simulink model "Control"  (R2025b)
settings: Solver=ode4  StartTime=0.0  StopTime=10.0  FixedStep=0.01  RelTol=1e-3
undefined symbols (not defined in the file): Control_Force_Limit, Control_phasing_power_threshold, Control_saturation_power_threshold, Control_switch, d_pulse_frequency, Dynamic_Nav_Gain, Dynamic_Navigation_constant, m_mass, Nav_constant, Phasing_switch, Pure_Pursuit_Centered_angle_Z, Pure_Pursuit_Y_Gain, Pure_Pursuit_Z_Gain, Ref_speed, s_energy_threshold
libraries: simulink x3
settings Model: DataDictionary=Control_data.sldd  Creator=mauro  LastModifiedBy=mauro

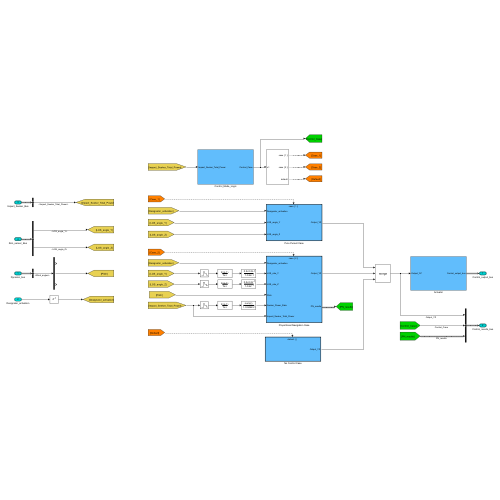
[thumbnail: Simulink's stored preview of the top-level diagram]
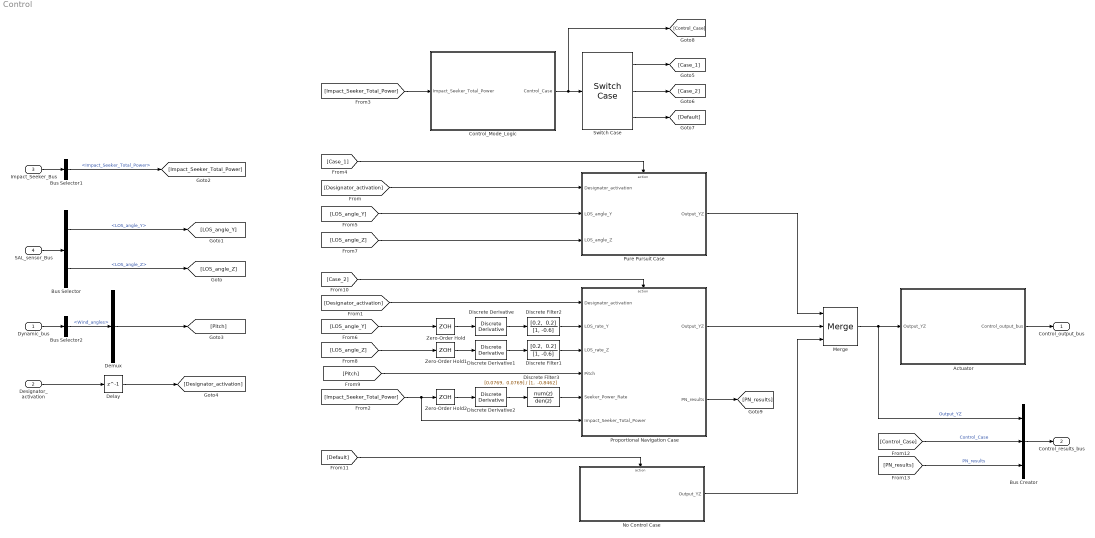
== system Control ==
  Dynamic_bus : Inport  OutDataTypeStr=Bus: Dynamic_bus
  Designator_activation : Inport  Port=2  OutDataTypeStr=double  SampleTime=0.01
  Impact_Seeker_Bus : Inport  Port=3  OutDataTypeStr=Bus: Impact_Seeker_Bus  BusOutputAsStruct=on
  SAL_sensor_Bus : Inport  Port=4  OutDataTypeStr=Bus: SAL_sensor_Bus  SampleTime=0.01  BusOutputAsStruct=on
  Actuator : Subsystem
  Bus Creator : BusCreator  Inputs=3  OutDataTypeStr=Bus: Control_results_bus  NonVirtualBus=on
  Bus Selector : BusSelector  OutputSignals=LOS_angle_Y,LOS_angle_Z
  Bus Selector1 : BusSelector  OutputSignals=Impact_Seeker_Total_Power
  Bus Selector2 : BusSelector  OutputSignals=Wind_angles
  Control_Mode_Logic : Subsystem
  Delay : Delay  DelayLength=1  InitialCondition=0
  Demux : Demux  Outputs=3
  Discrete Derivative : simulink/Discrete/Discrete Derivative  gainval=1.0  ICPrevScaledInput=0.0  OutMin=[]  OutMax=[]  OutDataType=fixdt(1, 16)  OutScaling=2^-10  DoSatur=off
  Discrete Derivative1 : simulink/Discrete/Discrete Derivative  gainval=1.0  ICPrevScaledInput=0  OutMin=[]  OutMax=[]  OutDataType=fixdt(1, 16)  OutScaling=2^-10  DoSatur=off
  Discrete Derivative2 : simulink/Discrete/Discrete Derivative  gainval=1.0  ICPrevScaledInput=0  OutMin=[]  OutMax=[]  OutDataType=fixdt(1, 16)  OutScaling=2^-10  DoSatur=off
  Discrete Filter1 : DiscreteFilter  Numerator="[0.2,  0.2]"  Denominator=[1, -0.6]
  Discrete Filter2 : DiscreteFilter  Numerator="[0.2,  0.2]"  Denominator=[1, -0.6]
  Discrete Filter3 : DiscreteFilter  Numerator="[0.0769,  0.0769]"  Denominator="[1,  -0.8462]"
  Merge : Merge  Inputs=3  InitialOutput=[0 0]
  No Control Case : Subsystem  TreatAsAtomicUnit=on
  Proportional Navigation Case : Subsystem  TreatAsAtomicUnit=on
  Pure Pursuit Case : Subsystem  TreatAsAtomicUnit=on
  Switch Case : SwitchCase  CaseConditions={1,2}
  Zero-Order Hold : ZeroOrderHold  SampleTime=1/d_pulse_frequency
  Zero-Order Hold1 : ZeroOrderHold  SampleTime=1/d_pulse_frequency
  Zero-Order Hold2 : ZeroOrderHold  SampleTime=1/d_pulse_frequency
  Control_output_bus : Outport  OutDataTypeStr=Bus: Control_output_bus  BusOutputAsStruct=on
  Control_results_bus : Outport  Port=2  OutDataTypeStr=Bus: Control_results_bus  BusOutputAsStruct=on
  wires:
  SAL_sensor_Bus/1 -> Bus Selector/1
  Bus Selector/2 -> [LOS_angle_Z]  "<LOS_angle_Z>"
  Bus Selector/1 -> [LOS_angle_Y]  "<LOS_angle_Y>"
  Dynamic_bus/1 -> Bus Selector2/1
  Bus Selector2/1 -> Demux/1  "<Wind_angles>"
  Actuator/1(Control_output_bus) -> Control_output_bus/1
  [Designator_activation] -> Pure Pursuit Case/1(Designator_activation)
  [Designator_activation] -> Proportional Navigation Case/1(Designator_activation)
  [LOS_angle_Y] -> Pure Pursuit Case/2(LOS_angle_Y)
  [LOS_angle_Z] -> Pure Pursuit Case/3(LOS_angle_Z)
  [Pitch] -> Proportional Navigation Case/4(Pitch)
  Proportional Navigation Case/1(Output_YZ) -> Merge/2
  Pure Pursuit Case/1(Output_YZ) -> Merge/1
  No Control Case/1(Output_YZ) -> Merge/3
  Merge/1 -> Bus Creator/1, Actuator/1(Output_YZ)  "Output_YZ"
  Control_Mode_Logic/1(Control_Case) -> [Control_Case], Switch Case/1
  Demux/2 -> [Pitch]
  Delay/1 -> [Designator_activation]
  Designator_activation/1 -> Delay/1
  [LOS_angle_Z] -> Zero-Order Hold1/1
  Discrete Derivative/1 -> Discrete Filter2/1
  Zero-Order Hold/1 -> Discrete Derivative/1
  [LOS_angle_Y] -> Zero-Order Hold/1
  Zero-Order Hold1/1 -> Discrete Derivative1/1
  Discrete Derivative1/1 -> Discrete Filter1/1
  Discrete Filter1/1 -> Proportional Navigation Case/3(LOS_rate_Z)
  Discrete Filter2/1 -> Proportional Navigation Case/2(LOS_rate_Y)
  Impact_Seeker_Bus/1 -> Bus Selector1/1
  Bus Selector1/1 -> [Impact_Seeker_Total_Power]  "<Impact_Seeker_Total_Power>"
  [Impact_Seeker_Total_Power] -> Control_Mode_Logic/1(Impact_Seeker_Total_Power)
  Zero-Order Hold2/1 -> Discrete Derivative2/1
  [Impact_Seeker_Total_Power] -> Zero-Order Hold2/1, Proportional Navigation Case/6(Impact_Seeker_Total_Power)
  Bus Creator/1 -> Control_results_bus/1
  Switch Case/1 -> [Case_1]
  Switch Case/2 -> [Case_2]
  Switch Case/3 -> [Default]
  [Case_1] -> Pure Pursuit Case/Action
  [Case_2] -> Proportional Navigation Case/Action
  [Default] -> No Control Case/Action
  Proportional Navigation Case/2(PN_results) -> [PN_results]
  [PN_results] -> Bus Creator/3  "PN_results"
  [Control_Case] -> Bus Creator/2  "Control_Case"
  Discrete Derivative2/1 -> Discrete Filter3/1
  Discrete Filter3/1 -> Proportional Navigation Case/5(Seeker_Power_Rate)

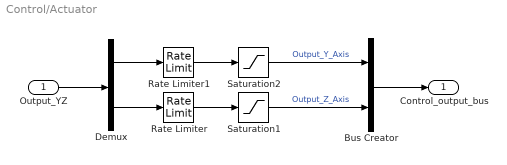
== system Control/Actuator ==
  Output_YZ : Inport
  Bus Creator : BusCreator  Inputs=2
  Demux : Demux  Outputs=2
  Rate Limiter : RateLimiter  RisingSlewLimit=1000  FallingSlewLimit=-1000  SampleTimeMode=inherited
  Rate Limiter1 : RateLimiter  RisingSlewLimit=2000  FallingSlewLimit=-2000  SampleTimeMode=inherited
  Saturation1 : Saturate  UpperLimit=Control_Force_Limit  LowerLimit=-Control_Force_Limit
  Saturation2 : Saturate  UpperLimit=Control_Force_Limit  LowerLimit=-Control_Force_Limit
  Control_output_bus : Outport  OutDataTypeStr=Bus: Control_output_bus
  wires:
  Saturation2/1 -> Bus Creator/1  "Output_Y_Axis"
  Rate Limiter1/1 -> Saturation2/1
  Output_YZ/1 -> Demux/1
  Saturation1/1 -> Bus Creator/2  "Output_Z_Axis"
  Bus Creator/1 -> Control_output_bus/1
  Rate Limiter/1 -> Saturation1/1
  Demux/1 -> Rate Limiter1/1
  Demux/2 -> Rate Limiter/1

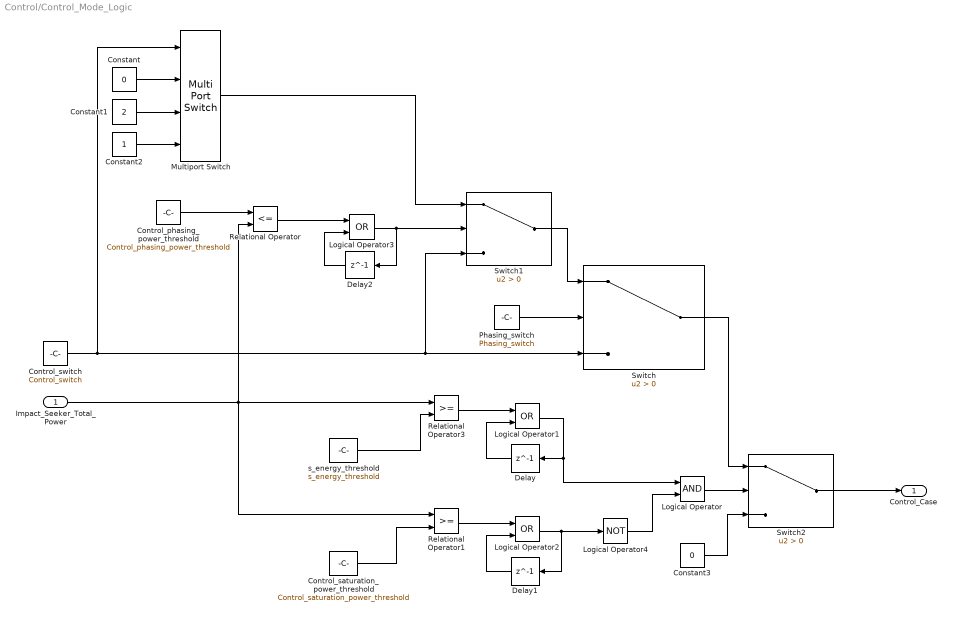
== system Control/Control_Mode_Logic ==
  Impact_Seeker_Total_Power : Inport
  Constant : Constant  Value=0
  Constant1 : Constant  Value=2
  Constant2 : Constant
  Constant3 : Constant  Value=0
  Control_phasing_power_threshold : Constant  Value=Control_phasing_power_threshold
  Control_saturation_power_threshold : Constant  Value=Control_saturation_power_threshold
  Control_switch : Constant  Value=Control_switch
  Delay : Delay  DelayLength=1  InitialCondition=0
  Delay1 : Delay  DelayLength=1  InitialCondition=0
  Delay2 : Delay  DelayLength=1  InitialCondition=0
  Logical Operator : Logic  AllPortsSameDT=off  OutDataTypeStr=boolean
  Logical Operator1 : Logic  Operator=OR  AllPortsSameDT=off  OutDataTypeStr=boolean
  Logical Operator2 : Logic  Operator=OR  AllPortsSameDT=off  OutDataTypeStr=boolean
  Logical Operator3 : Logic  Operator=OR  AllPortsSameDT=off  OutDataTypeStr=boolean
  Logical Operator4 : Logic  Operator=NOT  AllPortsSameDT=off  OutDataTypeStr=boolean
  Multiport Switch : MultiPortSwitch  DataPortOrder=Zero-based contiguous  zeroidx=on  SaturateOnIntegerOverflow=off  InputSameDT=off
  Phasing_switch : Constant  Value=Phasing_switch
  Relational Operator : RelationalOperator  Operator=<=  OutDataTypeStr=boolean  RndMeth=Simplest  InputSameDT=off
  Relational Operator1 : RelationalOperator  OutDataTypeStr=boolean  RndMeth=Simplest  InputSameDT=off
  Relational Operator3 : RelationalOperator  OutDataTypeStr=boolean  RndMeth=Simplest  InputSameDT=off
  Switch : Switch  Criteria=u2 > Threshold  SaturateOnIntegerOverflow=off  InputSameDT=off
  Switch1 : Switch  Criteria=u2 > Threshold  SaturateOnIntegerOverflow=off  InputSameDT=off
  Switch2 : Switch  Criteria=u2 > Threshold  SaturateOnIntegerOverflow=off  InputSameDT=off
  s_energy_threshold : Constant  Value=s_energy_threshold
  Control_Case : Outport
  wires:
  Control_switch/1 -> Switch/3, Switch1/3, Multiport Switch/1
  Switch1/1 -> Switch/1
  s_energy_threshold/1 -> Relational Operator3/2
  Phasing_switch/1 -> Switch/2
  Control_phasing_power_threshold/1 -> Relational Operator/1
  Switch/1 -> Switch2/1
  Constant3/1 -> Switch2/3
  Constant/1 -> Multiport Switch/2
  Constant2/1 -> Multiport Switch/4
  Multiport Switch/1 -> Switch1/1
  Constant1/1 -> Multiport Switch/3
  Switch2/1 -> Control_Case/1
  Logical Operator1/1 -> Logical Operator/1, Delay/1
  Relational Operator3/1 -> Logical Operator1/1
  Delay/1 -> Logical Operator1/2
  Logical Operator2/1 -> Delay1/1, Logical Operator4/1
  Delay1/1 -> Logical Operator2/2
  Relational Operator1/1 -> Logical Operator2/1
  Logical Operator3/1 -> Delay2/1, Switch1/2
  Delay2/1 -> Logical Operator3/2
  Relational Operator/1 -> Logical Operator3/1
  Control_saturation_power_threshold/1 -> Relational Operator1/2
  Logical Operator/1 -> Switch2/2
  Logical Operator4/1 -> Logical Operator/2
  Impact_Seeker_Total_Power/1 -> Relational Operator3/1, Relational Operator1/1, Relational Operator/2

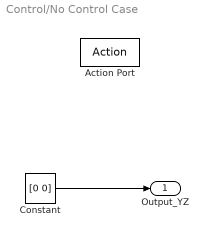
== system Control/No Control Case ==
  Action Port : ActionPort  ActionPortLabel=default:
  Constant : Constant  Value=[0 0]
  Output_YZ : Outport
  wires:
  Constant/1 -> Output_YZ/1

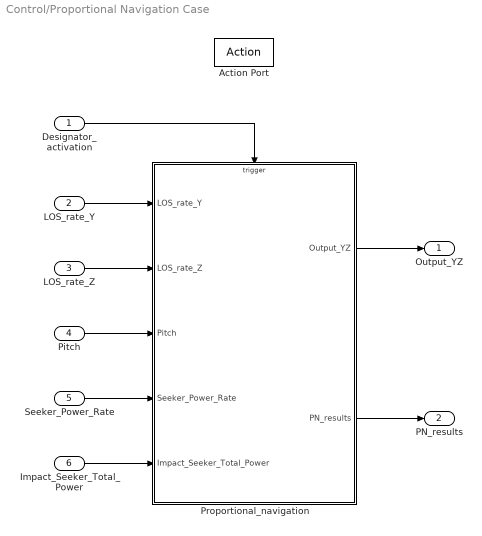
== system Control/Proportional Navigation Case ==
  Designator_activation : Inport
  LOS_rate_Y : Inport  Port=2
  LOS_rate_Z : Inport  Port=3
  Pitch : Inport  Port=4
  Seeker_Power_Rate : Inport  Port=5
  Impact_Seeker_Total_Power : Inport  Port=6
  Action Port : ActionPort  ActionPortLabel=case [ 2 ]:
  Proportional_navigation : Subsystem
  Output_YZ : Outport
  PN_results : Outport  Port=2  OutDataTypeStr=Bus: PN_results_bus
  wires:
  Proportional_navigation/1(Output_YZ) -> Output_YZ/1
  Pitch/1 -> Proportional_navigation/3(Pitch)
  Designator_activation/1 -> Proportional_navigation/Trigger
  LOS_rate_Z/1 -> Proportional_navigation/2(LOS_rate_Z)
  LOS_rate_Y/1 -> Proportional_navigation/1(LOS_rate_Y)
  Seeker_Power_Rate/1 -> Proportional_navigation/4(Seeker_Power_Rate)
  Impact_Seeker_Total_Power/1 -> Proportional_navigation/5(Impact_Seeker_Total_Power)
  Proportional_navigation/2(PN_results) -> PN_results/1

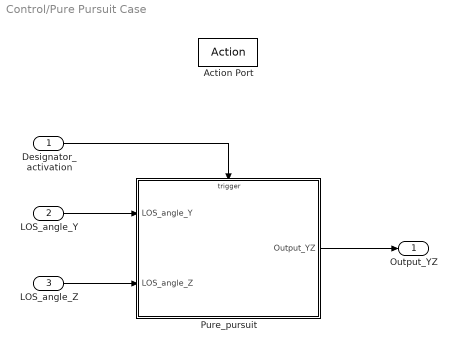
== system Control/Pure Pursuit Case ==
  Designator_activation : Inport
  LOS_angle_Y : Inport  Port=2
  LOS_angle_Z : Inport  Port=3
  Action Port : ActionPort  ActionPortLabel=case [ 1 ]:
  Pure_pursuit : Subsystem
  Output_YZ : Outport
  wires:
  LOS_angle_Z/1 -> Pure_pursuit/2(LOS_angle_Z)
  LOS_angle_Y/1 -> Pure_pursuit/1(LOS_angle_Y)
  Pure_pursuit/1(Output_YZ) -> Output_YZ/1
  Designator_activation/1 -> Pure_pursuit/Trigger

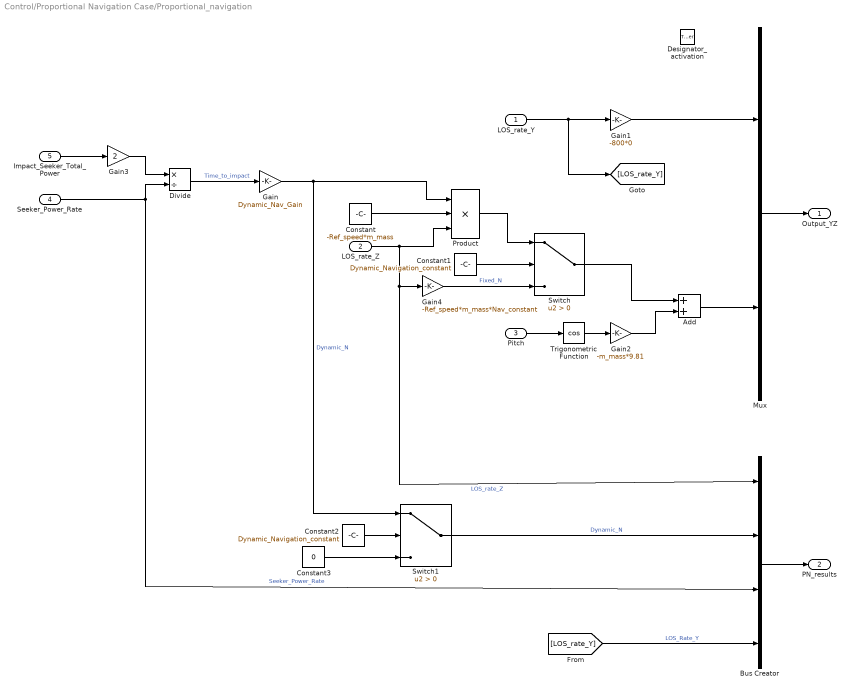
== system Control/Proportional Navigation Case/Proportional_navigation ==
  LOS_rate_Y : Inport
  LOS_rate_Z : Inport  Port=2
  Pitch : Inport  Port=3
  Seeker_Power_Rate : Inport  Port=4
  Impact_Seeker_Total_Power : Inport  Port=5
  Designator_activation : TriggerPort  VariantControl=(inherit)  PortDimensions=1
  Add : Sum
  Bus Creator : BusCreator  Inputs=4  OutDataTypeStr=Bus: PN_results_bus  NonVirtualBus=on
  Constant : Constant  Value=-Ref_speed*m_mass
  Constant1 : Constant  Value=Dynamic_Navigation_constant
  Constant2 : Constant  Value=Dynamic_Navigation_constant
  Constant3 : Constant  Value=0
  Divide : Product  Inputs=*/
  Gain : Gain  Gain=Dynamic_Nav_Gain
  Gain1 : Gain  Gain=-800*0
  Gain2 : Gain  Gain=-m_mass*9.81
  Gain3 : Gain  Gain=2
  Gain4 : Gain  Gain=-Ref_speed*m_mass*Nav_constant
  Mux : Mux  Inputs=2
  Product : Product  Inputs=3
  Switch : Switch  Criteria=u2 > Threshold  SaturateOnIntegerOverflow=off  InputSameDT=off
  Switch1 : Switch  Criteria=u2 > Threshold  SaturateOnIntegerOverflow=off  InputSameDT=off
  Trigonometric Function : Trigonometry  Operator=cos
  Output_YZ : Outport  OutputWhenDisabled=reset  InitialOutput=[0 0]
  PN_results : Outport  Port=2  OutDataTypeStr=Bus: PN_results_bus  OutputWhenDisabled=reset  InitialOutput=0
  wires:
  Mux/1 -> Output_YZ/1
  LOS_rate_Y/1 -> [LOS_rate_Y], Gain1/1
  Pitch/1 -> Trigonometric Function/1
  Trigonometric Function/1 -> Gain2/1
  Gain2/1 -> Add/2
  Gain1/1 -> Mux/1
  Impact_Seeker_Total_Power/1 -> Gain3/1
  Seeker_Power_Rate/1 -> Bus Creator/3, Divide/2  "Seeker_Power_Rate"
  Gain3/1 -> Divide/1
  Divide/1 -> Gain/1  "Time_to_impact"
  LOS_rate_Z/1 -> Product/3, Bus Creator/1, Gain4/1  "LOS_rate_Z"
  Constant/1 -> Product/2
  Gain/1 -> Switch1/1, Product/1  "Dynamic_N"
  Product/1 -> Switch/1
  Constant1/1 -> Switch/2
  Gain4/1 -> Switch/3  "Fixed_N"
  Switch/1 -> Add/1
  Bus Creator/1 -> PN_results/1
  [LOS_rate_Y] -> Bus Creator/4  "LOS_Rate_Y"
  Add/1 -> Mux/2
  Switch1/1 -> Bus Creator/2  "Dynamic_N"
  Constant2/1 -> Switch1/2
  Constant3/1 -> Switch1/3

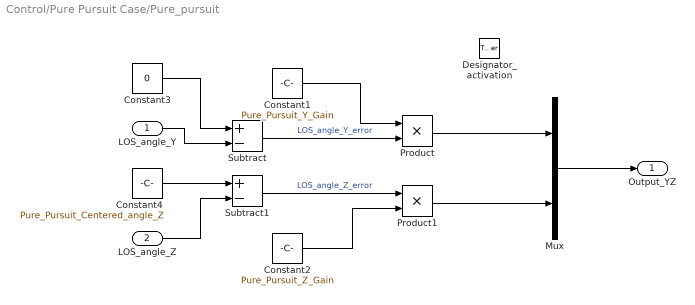
== system Control/Pure Pursuit Case/Pure_pursuit ==
  LOS_angle_Y : Inport
  LOS_angle_Z : Inport  Port=2
  Designator_activation : TriggerPort  VariantControl=(inherit)  PortDimensions=1
  Constant1 : Constant  Value=Pure_Pursuit_Y_Gain
  Constant2 : Constant  Value=Pure_Pursuit_Z_Gain
  Constant3 : Constant  Value=0
  Constant4 : Constant  Value=Pure_Pursuit_Centered_angle_Z
  Mux : Mux  Inputs=2
  Product : Product
  Product1 : Product
  Subtract : Sum  Inputs=+-
  Subtract1 : Sum  Inputs=+-
  Output_YZ : Outport
  wires:
  Constant2/1 -> Product1/2
  Constant1/1 -> Product/1
  LOS_angle_Y/1 -> Subtract/2
  Constant3/1 -> Subtract/1
  Subtract1/1 -> Product1/1  "LOS_angle_Z_error"
  Subtract/1 -> Product/2  "LOS_angle_Y_error"
  LOS_angle_Z/1 -> Subtract1/2
  Mux/1 -> Output_YZ/1
  Product/1 -> Mux/1
  Constant4/1 -> Subtract1/1
  Product1/1 -> Mux/2
